simulink model "bloques_rodadura1y2"  (R2015b)
settings: Solver=ode45  StartTime=0  StopTime=1000  FixedStep=0.001  RelTol=1e-3
libraries: simulink_extras x7, aerolibtransform2 x2, aerolibutil x2, simulink x1, aerolibobsolete x1, aerolibfltsims x1, aerolibasang x1
(part 2 of 2)

== system bloques_rodadura1y2/Planta/Forces and Moments in Take-off/Transition/Aerodynamic Moments /Roll Moment/Roll Moment Coefficient ==
  "beta " : Inport
  delta_a : Inport  Port=2
  delta_r : Inport  Port=3
  C_l0 : Constant  Value=0
  C_lbeta : Constant  Value=-0.0895
  C_ldelta_a : Constant  Value=0.2290
  C_ldelta_r : Constant  Value=0.0147
  Product1 : Product
  Product2 : Product
  Product3 : Product
  "Sum " : Sum  Inputs=++++
  C_l : Outport
  wires:
  "beta "/1 -> Product1/1
  C_lbeta/1 -> Product1/2
  delta_a/1 -> Product2/1
  C_ldelta_a/1 -> Product2/2
  delta_r/1 -> Product3/1
  C_ldelta_r/1 -> Product3/2
  C_l0/1 -> "Sum "/1
  Product1/1 -> "Sum "/2
  Product2/1 -> "Sum "/3
  Product3/1 -> "Sum "/4
  "Sum "/1 -> C_l/1

== system bloques_rodadura1y2/Planta/Forces and Moments in Take-off/Transition/Aerodynamic Moments /Yaw Moment/Dynamic pressure  ==
  V : Inport
  "rho " : Inport  Port=2
  Constant : Constant  Value=0.5
  Math Function : Math  Operator=square  SaturateOnIntegerOverflow=on
  Product : Product  Inputs=3
  q : Outport
  wires:
  Math Function/1 -> Product/1
  "rho "/1 -> Product/3
  Product/1 -> q/1
  Constant/1 -> Product/2
  V/1 -> Math Function/1

== system bloques_rodadura1y2/Planta/Forces and Moments in Take-off/Transition/Aerodynamic Moments /Yaw Moment/Yaw Moment Coefficient ==
  "beta " : Inport
  delta_a : Inport  Port=2
  delta_r : Inport  Port=3
  C_n0 : Constant  Value=0
  C_nbeta : Constant  Value=0.0907
  C_ndelta_a : Constant  Value=-0.0504
  C_ndelta_r : Constant  Value=-0.0805
  Product1 : Product
  Product2 : Product
  Product3 : Product
  "Sum " : Sum  Inputs=++++
  C_n : Outport
  wires:
  "beta "/1 -> Product1/1
  C_nbeta/1 -> Product1/2
  delta_a/1 -> Product2/1
  C_ndelta_a/1 -> Product2/2
  delta_r/1 -> Product3/1
  C_ndelta_r/1 -> Product3/2
  C_n0/1 -> "Sum "/1
  Product1/1 -> "Sum "/2
  Product2/1 -> "Sum "/3
  Product3/1 -> "Sum "/4
  "Sum "/1 -> C_n/1
